simulink model "Lab_2"  (Simulink 9.2)
settings: Solver=ode45  StartTime=0.0  StopTime=simulation_time  RelTol=1e-10
values from neighbouring files (symbols this model uses):
  I = [I_1,   0,  0 ... (first row only)    [main.m]
  I_inv = inv(I)    [main.m]
  w_0 = [w1_0, w2_0, w3_0]    [main.m]
undefined symbols (not defined in the file or in its folder): DCM_0, k_11, k_12, k_21, k_22, phi_0, phi_d, psi_0, psi_d, theta_0, theta_d
libraries: sharedutil x1
settings Model: Creator=fcuzzocrea  LastModifiedBy=fcuzzocrea
settings DataIOCC: LimitDataPoints=off  SaveFormat=Dataset  SignalLoggingSaveFormat=Dataset
settings OptimizationCC: LifeSpan=auto
settings DebuggingCC: UnderspecifiedInitializationDetection=Simplified  MergeDetectMultiDrivingBlocksExec=error  FcnCallInpInsideContextMsg=error  StateNameClashWarn=none  LibraryContextMissingDiagnostic=none  SFUnexpectedBacktrackingDiag=error  SFNoUnconditionalDefaultTransitionDiag=error  SFExecutionAtInitializationDiag=warning
settings HardwareCC: ProdBitPerPointer=64  ProdBitPerSizeT=64  ProdBitPerPtrDiffT=64  ProdLargestAtomicFloat=Float  ProdIntDivRoundTo=Zero  ProdEndianess=LittleEndian  ProdWordSize=64  ProdHWDeviceType=Intel->x86-64 (Windows64)
settings ModelReferenceCC: PropagateSignalLabelsOutOfModel=on
settings CodeAppCC: StateflowObjectComments=off
settings GRTTargetCC: TargetLangStandard=C99 (ISO)  GeneratePreprocessorConditionals=Use local settings  CombineOutputUpdateFcns=on  GRTInterface=off
settings ConfigComp: CovMetricSettings=dwe  CovHtmlReporting=off  CovSaveCumulativeToWorkspaceVar=off  CovSaveSingleToWorkspaceVar=off  CovExternalEMLEnable=on

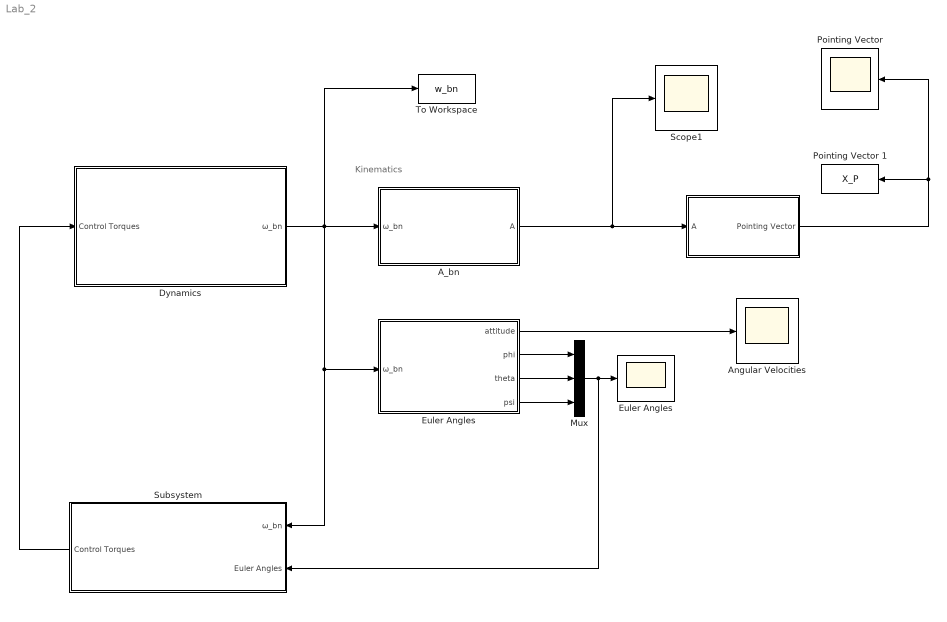
== system Lab_2 ==
  note: Kinematics
  " " : Subsystem
  A_bn : Subsystem
  "Angular Velocities " : Scope
  "Dynamics  " : Subsystem
  Euler Angles : Scope
  "Euler Angles " : Subsystem
  Mux : Mux  Inputs=3
  Pointing Vector : Scope
  Pointing Vector 1 : ToWorkspace  VariableName=X_P  SampleTime=-1
  Scope1 : Scope
  Subsystem : Subsystem
  To Workspace : ToWorkspace  VariableName=w_bn  SampleTime=-1
  wires:
  A_bn/1(A) -> Scope1/1, " "/1(A)
  "Euler Angles "/1(attitude) -> "Angular Velocities "/1
  "Dynamics  "/1(ω_bn) -> Subsystem/1(ω_bn), "Euler Angles "/1(ω_bn), To Workspace/1, A_bn/1(ω_bn)
  " "/1("Pointing Vector ") -> Pointing Vector/1, Pointing Vector 1/1
  "Euler Angles "/2(phi) -> Mux/1
  "Euler Angles "/3(theta) -> Mux/2
  "Euler Angles "/4(psi) -> Mux/3
  Mux/1 -> Subsystem/2(Euler Angles), Euler Angles/1
  Subsystem/1(Control Torques) -> "Dynamics  "/1(Control Torques)

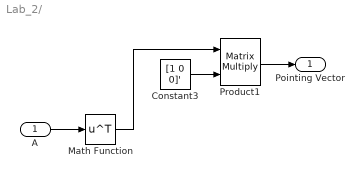
== system Lab_2/  ==
  A : Inport
  Constant3 : Constant  Value=[1 0 0]'  VectorParams1D=off
  Math Function : Math  Operator=transpose  SaturateOnIntegerOverflow=on
  Product1 : Product  Multiplication=Matrix(*)
  "Pointing Vector " : Outport
  wires:
  Constant3/1 -> Product1/2
  Math Function/1 -> Product1/1
  A/1 -> Math Function/1
  Product1/1 -> "Pointing Vector "/1

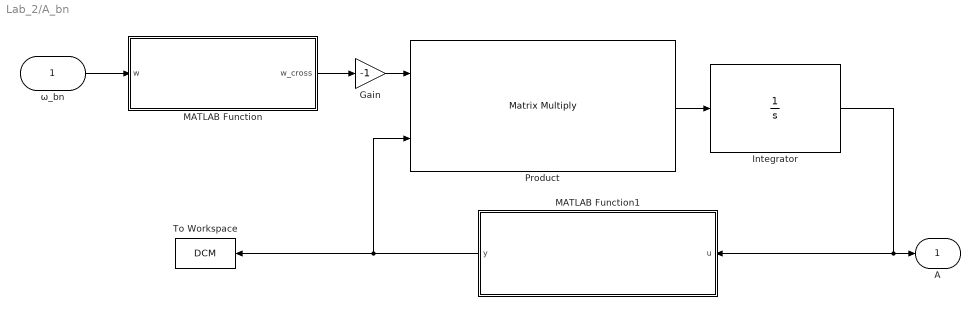
== system Lab_2/A_bn ==
  ω_bn : Inport  Unit=rad/s  PortDimensions=3
  Gain : Gain  Gain=-1
  Integrator : Integrator  InitialCondition=DCM_0
  MATLAB Function : MATLAB Function  TreatAsAtomicUnit=on
  MATLAB Function1 : MATLAB Function  TreatAsAtomicUnit=on
  Product : Product  Multiplication=Matrix(*)
  To Workspace : ToWorkspace  VariableName=DCM  SampleTime=-1
  A : Outport
  wires:
  Product/1 -> Integrator/1
  MATLAB Function/1(w_cross) -> Gain/1
  Integrator/1 -> MATLAB Function1/1(u), A/1
  ω_bn/1 -> MATLAB Function/1(w)
  Gain/1 -> Product/1
  MATLAB Function1/1(y) -> Product/2, To Workspace/1

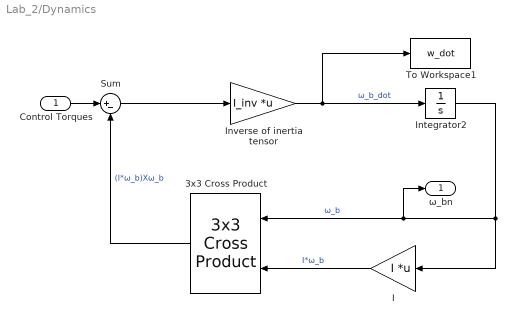
== system Lab_2/Dynamics   ==
  Control Torques : Inport
  3x3 Cross Product : sharedutil/3x3 Cross Product  aMode=aMode
      settings: SourceProductBaseCode=AE
  I : Gain  Gain=I  Multiplication=Matrix(K*u)
  Integrator2 : Integrator  InitialCondition=w_0
  Inverse of inertia tensor : Gain  Gain=I_inv  Multiplication=Matrix(K*u)
  Sum : Sum  Inputs=|+-
  To Workspace1 : ToWorkspace  VariableName=w_dot  SampleTime=-1
  ω_bn : Outport
  wires:
  Integrator2/1 -> I/1, 3x3 Cross Product/1, ω_bn/1  "ω_b"
  Inverse of inertia tensor/1 -> To Workspace1/1, Integrator2/1  "ω_b_dot"
  I/1 -> 3x3 Cross Product/2  "I*ω_b"
  3x3 Cross Product/1 -> Sum/2  "(I*ω_b)Xω_b"
  Sum/1 -> Inverse of inertia tensor/1
  Control Torques/1 -> Sum/1

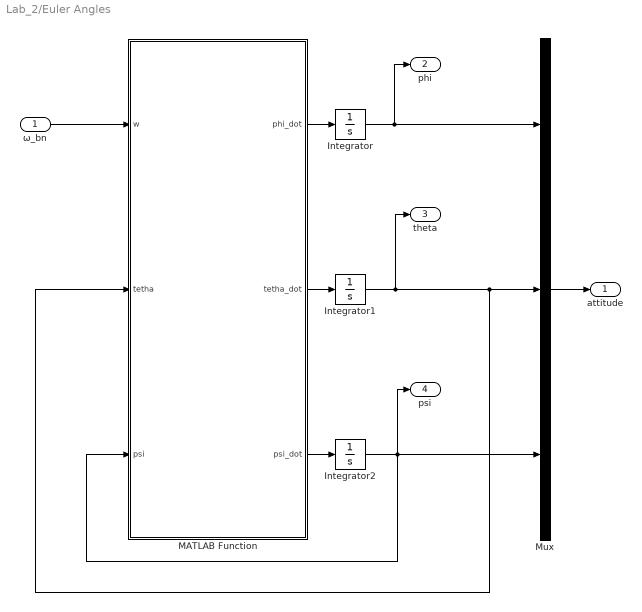
== system Lab_2/Euler Angles  ==
  ω_bn : Inport
  Integrator : Integrator  InitialCondition=phi_0
  Integrator1 : Integrator  InitialCondition=theta_0
  Integrator2 : Integrator  InitialCondition=psi_0
  MATLAB Function : MATLAB Function  TreatAsAtomicUnit=on
  Mux : Mux  Inputs=3
  attitude : Outport
  phi : Outport  Port=2
  theta : Outport  Port=3
  psi : Outport  Port=4
  wires:
  ω_bn/1 -> MATLAB Function/1(w)
  MATLAB Function/1(phi_dot) -> Integrator/1
  MATLAB Function/2(tetha_dot) -> Integrator1/1
  MATLAB Function/3(psi_dot) -> Integrator2/1
  Integrator/1 -> phi/1, Mux/1
  Integrator1/1 -> theta/1, Mux/2, MATLAB Function/2(tetha)
  Mux/1 -> attitude/1
  Integrator2/1 -> psi/1, Mux/3, MATLAB Function/3(psi)

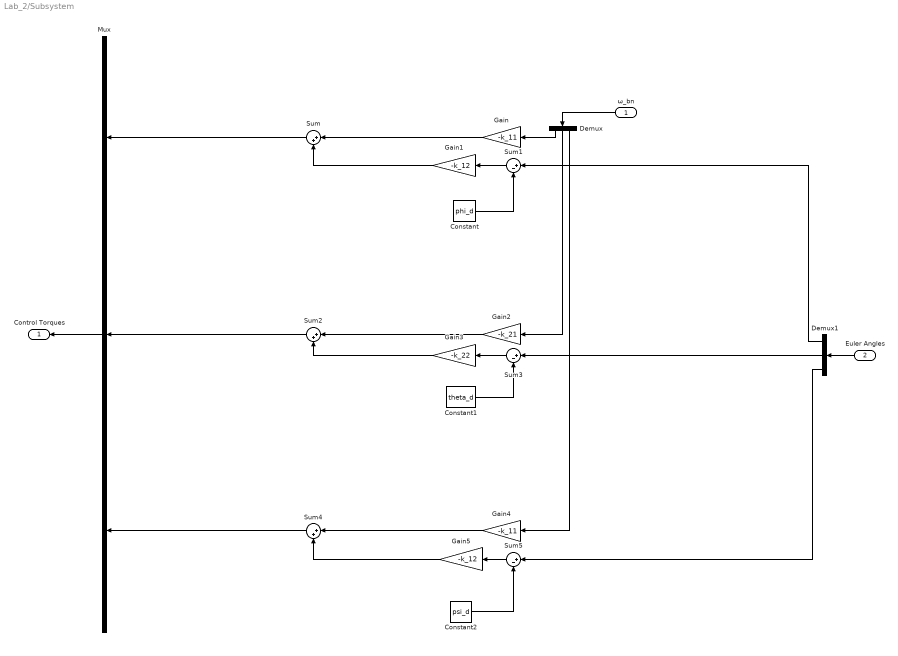
== system Lab_2/Subsystem ==
  ω_bn : Inport
  Euler Angles : Inport  Port=2
  Constant : Constant  Value=phi_d
  Constant1 : Constant  Value=theta_d
  Constant2 : Constant  Value=psi_d
  Demux : Demux  Outputs=3
  Demux1 : Demux  Outputs=3
  Gain : Gain  Gain=-k_11
  Gain1 : Gain  Gain=-k_12
  Gain2 : Gain  Gain=-k_21
  Gain3 : Gain  Gain=-k_22
  Gain4 : Gain  Gain=-k_11
  Gain5 : Gain  Gain=-k_12
  Mux : Mux  Inputs=3
  Sum : Sum  Inputs=|++
  Sum1 : Sum  Inputs=|+-
  Sum2 : Sum  Inputs=|++
  Sum3 : Sum  Inputs=|+-
  Sum4 : Sum  Inputs=|++
  Sum5 : Sum  Inputs=|+-
  Control Torques : Outport
  wires:
  Sum2/1 -> Mux/2
  Constant2/1 -> Sum5/2
  Demux1/2 -> Sum3/1
  Constant/1 -> Sum1/2
  Demux/2 -> Gain2/1
  Gain3/1 -> Sum2/2
  Gain5/1 -> Sum4/2
  Sum3/1 -> Gain3/1
  Sum5/1 -> Gain5/1
  Gain4/1 -> Sum4/1
  Sum1/1 -> Gain1/1
  Gain2/1 -> Sum2/1
  Euler Angles/1 -> Demux1/1
  Demux1/3 -> Sum5/1
  Sum4/1 -> Mux/3
  Gain/1 -> Sum/1
  Demux/3 -> Gain4/1
  ω_bn/1 -> Demux/1
  Constant1/1 -> Sum3/2
  Gain1/1 -> Sum/2
  Demux/1 -> Gain/1
  Demux1/1 -> Sum1/1
  Mux/1 -> Control Torques/1
  Sum/1 -> Mux/1

== matlab function Euler Angles /MATLAB Function ==
  data: phi_dot output double; tetha_dot output double; psi_dot output double; w input double; tetha input double; psi input double
function [phi_dot,tetha_dot, psi_dot] = euler_eqtns(w, tetha, psi)

% Euler rotations (sequence 123)
phi_dot = 1/cos(tetha)*((w(1)*cos(psi)-w(2)*sin(psi)));
tetha_dot = (w(2)*cos(psi))+(w(1)*sin(psi));
psi_dot = w(3) - ((w(1)*cos(psi) - w(2)*sin(psi))*(sin(tetha)/cos(tetha)));

end

== matlab function A_bn/MATLAB Function1 ==
  data: u input double; y output double
function y = ortonormalize(u)
%#codegen
% Ortonormalize a matrix.
% Reference : Lecture 7, Slide 5 SADC Polimi

y = u.*3/2 - u*u'*(u./2);

y = u;

end

== matlab function A_bn/MATLAB Function ==
  data: w input double; w_cross output double
function w_cross  = assembly_w_cross(w)

w_cross = [0, -w(3), w(2);
           w(3), 0, -w(1);
          -w(2), w(1), 0];
